simulink model "Model_simulink_passive_Torque"  (R2012b)
settings: Solver=ode3  SolverMode=SingleTasking  StartTime=0.0  StopTime=Tend  FixedStep=0.0001  RelTol=1e-3
undefined symbols (not defined in the file): In, J, Kp, Kt, Kw, Lambda, m, Mn, psi, Rt, T, TR, Un, Uz0, V, wn, Y
settings Model: Creator=user  LastModifiedBy=Adam
settings DataIOCC: SignalLoggingSaveFormat=ModelDataLogs
settings OptimizationCC: BlockReduction=off  BooleanDataType=off
settings DebuggingCC: SaveWithParameterizedLinksMsg=none  SignalResolutionControl=TryResolveAllWithWarning  SolverPrmCheckMsg=none  MultiTaskDSMMsg=warning  MultiTaskCondExecSysMsg=none  StrictBusMsg=None
settings HardwareCC: TargetUnknown=on
settings RTWCC: IncludeERTFirstTime=on

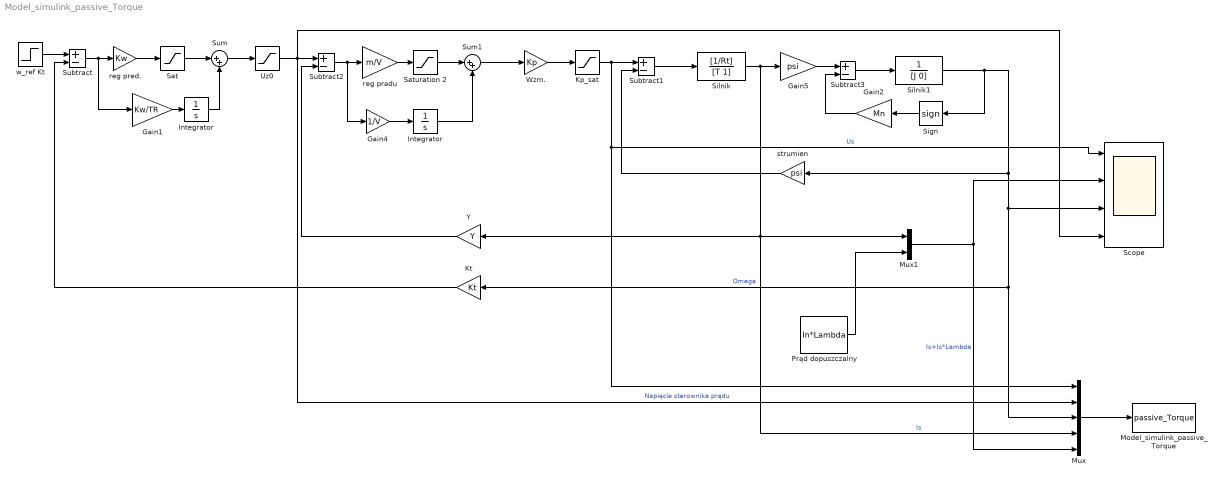
== system Model_simulink_passive_Torque ==
  Gain1 : Gain  Gain=Kw/TR
  Gain2 : Gain  Gain=Mn
  Gain4 : Gain  Gain=1/V
  Gain5 : Gain  Gain=psi
  Integrator : Integrator  LimitOutput=on  UpperSaturationLimit=10  LowerSaturationLimit=-10
  "Integrator " : Integrator  LimitOutput=on  UpperSaturationLimit=10  LowerSaturationLimit=-10
  Kp_sat : Saturate  UpperLimit=1.5*Un  LowerLimit=-1.5*Un
  Kt : Gain  Gain=Kt
  Model_simulink_passive_Torque : ToWorkspace  VariableName=passive_Torque  SampleTime=-1  SaveFormat=Structure With Time
  Mux : Mux  Inputs=5
  Mux1 : Mux  Inputs=2
  Prąd dopuszczalny : Constant  Value=In*Lambda
  Sat : Saturate  UpperLimit=10  LowerLimit=-10
  Saturation 2 : Saturate  UpperLimit=10  LowerLimit=-10
  Scope : Scope  NumInputPorts=4
      settings: TimeRange=10  YMin=3.15~0~-2e-07~9.36937  YMax=3.5~250~2.5e-07~10.3556
  Sign : Signum  ZeroCross=off
  Silnik : TransferFcn  Numerator=[1/Rt]  Denominator=[T 1]
  Silnik1 : TransferFcn  Numerator=1  Denominator=[J 0]
  Subtract{,1..3} (4 alike) : Sum  Inputs=+-
  Sum : Sum  Inputs=|++
  Sum1 : Sum  Inputs=|++
  Uz0 : Saturate  UpperLimit=Uz0  LowerLimit=-Uz0
  Wzm. : Gain  Gain=Kp
  Y : Gain  Gain=Y
  reg pradu : Gain  Gain=m/V
  reg pred. : Gain  Gain=Kw
  strumien : Gain  Gain=psi
  w_ref Kt : Step  Time=0  After=wn*Kt  SampleTime=0
  wires:
  w_ref Kt/1 -> Subtract/1
  Subtract/1 -> Gain1/1, reg pred./1
  Gain1/1 -> Integrator/1
  reg pradu/1 -> Saturation 2/1
  Wzm./1 -> Kp_sat/1
  Gain4/1 -> "Integrator "/1
  Subtract1/1 -> Silnik/1
  Silnik/1 -> Mux/4, Y/1, Mux1/1, Gain5/1  "Is"
  Gain5/1 -> Subtract3/1
  Subtract3/1 -> Silnik1/1
  strumien/1 -> Subtract1/2
  Kp_sat/1 -> Mux/1, Scope/1, Subtract1/1  "Us"
  Y/1 -> Subtract2/2
  Mux1/1 -> Mux/5, Scope/2  "Is+Is*Lambda"
  Prąd dopuszczalny/1 -> Mux1/2
  Uz0/1 -> Mux/2, Scope/4, Subtract2/1  "Napięcie sterownika prądu"
  Silnik1/1 -> Sign/1, Mux/3, Kt/1, Scope/3, strumien/1  "Omega"
  Kt/1 -> Subtract/2
  reg pred./1 -> Sat/1
  Saturation 2/1 -> Sum1/1
  Sum1/1 -> Wzm./1
  "Integrator "/1 -> Sum1/2
  Subtract2/1 -> Gain4/1, reg pradu/1
  Sat/1 -> Sum/1
  Sum/1 -> Uz0/1
  Integrator/1 -> Sum/2
  Mux/1 -> Model_simulink_passive_Torque/1
  Sign/1 -> Gain2/1
  Gain2/1 -> Subtract3/2
